simulink model "3DoFManipulator_SIMULATION"  (R2023b)
settings: Solver=ode45  StartTime=0.0  StopTime=10  RelTol=1e-3
undefined symbols (not defined in the file): X, Y, Z
libraries: sm_lib x10, nesl_utility x7, slpidlib x6, robotmaniplib x2
settings Model: Creator=nicog  LastModifiedBy=nicog

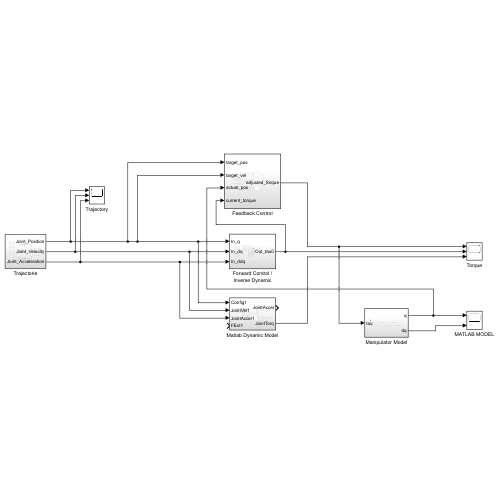
[thumbnail: Simulink's stored preview of the top-level diagram]
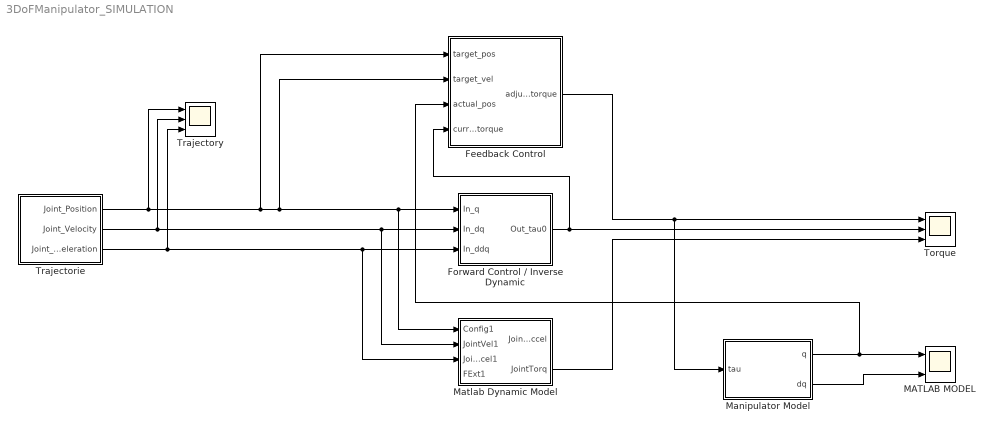
== system 3DoFManipulator_SIMULATION ==
  Feedback Control : Subsystem
  Forward Control / Inverse Dynamic : Subsystem
  MATLAB MODEL : Scope  NumInputPorts=2
  Manipulator Model : Subsystem
  Matlab Dynamic Model : Subsystem
  Torque : Scope  NumInputPorts=3
  Trajectorie : Subsystem
  Trajectory : Scope  NumInputPorts=3
  wires:
  Trajectorie/2(Joint_Velocity) -> Forward Control / Inverse Dynamic/2(In_dq), Matlab Dynamic Model/2(JointVel1), Trajectory/2
  Trajectorie/1(Joint_Position) -> Trajectory/1, Feedback Control/1(target_pos), Feedback Control/2(target_vel), Forward Control / Inverse Dynamic/1(In_q), Matlab Dynamic Model/1(Config1)
  Matlab Dynamic Model/2(JointTorq) -> Torque/3
  Trajectorie/3(Joint_Acceleration) -> Forward Control / Inverse Dynamic/3(In_ddq), Matlab Dynamic Model/3(JointAccel1), Trajectory/3
  Forward Control / Inverse Dynamic/1(Out_tau0) -> Feedback Control/4(current_torque), Torque/2
  Manipulator Model/1(q) -> Feedback Control/3(actual_pos), MATLAB MODEL/1
  Feedback Control/1(adjusted_torque) -> Manipulator Model/1(tau), Torque/1
  Manipulator Model/2(dq) -> MATLAB MODEL/2

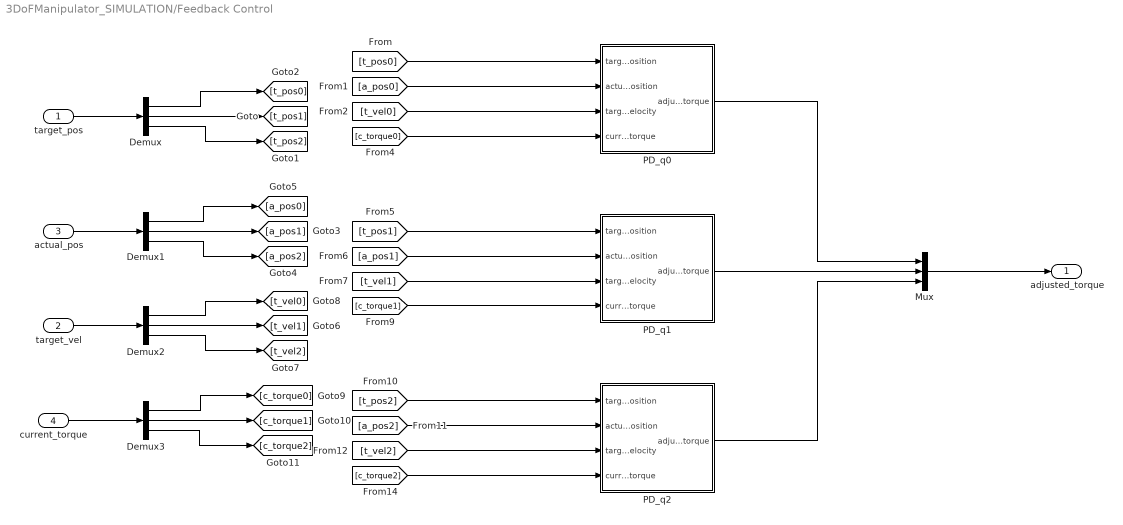
== system 3DoFManipulator_SIMULATION/Feedback Control ==
  target_pos : Inport
  target_vel : Inport  Port=2
  actual_pos : Inport  Port=3
  current_torque : Inport  Port=4
  Demux{,1..3} (4 alike) : Demux  Outputs=3
  Mux : Mux  Inputs=3
  PD_q0 : Subsystem
  PD_q1 : Subsystem
  PD_q2 : Subsystem
  adjusted_torque : Outport
  wires:
  target_pos/1 -> Demux/1
  actual_pos/1 -> Demux1/1
  target_vel/1 -> Demux2/1
  Demux/1 -> [t_pos0]
  Demux/2 -> [t_pos1]
  Demux/3 -> [t_pos2]
  Demux1/1 -> [a_pos0]
  Demux1/2 -> [a_pos1]
  Demux1/3 -> [a_pos2]
  Demux2/1 -> [t_vel0]
  Demux2/2 -> [t_vel1]
  Demux2/3 -> [t_vel2]
  [t_pos0] -> PD_q0/1(target position)
  [a_pos0] -> PD_q0/2(actual position)
  [t_vel0] -> PD_q0/3(target velocity)
  [c_torque0] -> PD_q0/4(current torque)
  Mux/1 -> adjusted_torque/1
  [c_torque1] -> PD_q1/4(current torque)
  [a_pos1] -> PD_q1/2(actual position)
  [t_vel1] -> PD_q1/3(target velocity)
  [t_pos1] -> PD_q1/1(target position)
  [c_torque2] -> PD_q2/4(current torque)
  [a_pos2] -> PD_q2/2(actual position)
  [t_vel2] -> PD_q2/3(target velocity)
  [t_pos2] -> PD_q2/1(target position)
  PD_q1/1(adjusted_torque) -> Mux/2
  PD_q2/1(adjusted_torque) -> Mux/3
  current_torque/1 -> Demux3/1
  Demux3/1 -> [c_torque0]
  Demux3/2 -> [c_torque1]
  Demux3/3 -> [c_torque2]
  PD_q0/1(adjusted_torque) -> Mux/1

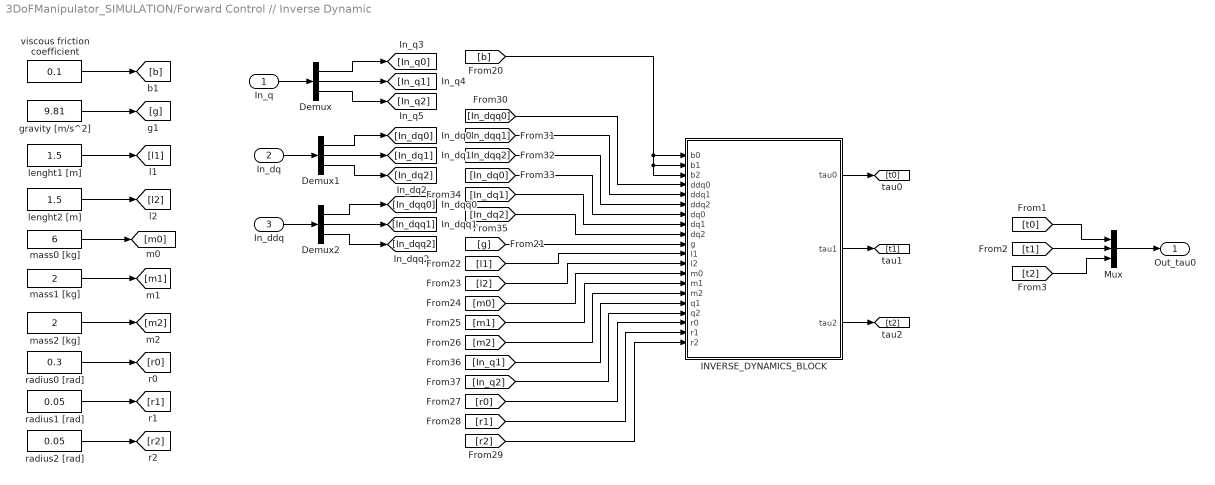
== system 3DoFManipulator_SIMULATION/Forward Control // Inverse Dynamic ==
  In_q : Inport
  In_dq : Inport  Port=2
  In_ddq : Inport  Port=3
  Demux : Demux  Outputs=3
  Demux1 : Demux  Outputs=3
  Demux2 : Demux  Outputs=3
  INVERSE_DYNAMICS_BLOCK : MATLAB Function  TreatAsAtomicUnit=on
  Mux : Mux  Inputs=3
  "gravity [m/s^2] " : Constant  Value=9.81
  lenght1 [m] : Constant  Value=1.5
  lenght2 [m] : Constant  Value=1.5
  mass0 [kg] : Constant  Value=6
  mass1 [kg] : Constant  Value=2
  mass2 [kg] : Constant  Value=2
  radius0 [rad] : Constant  Value=0.3
  radius1 [rad] : Constant  Value=0.05
  radius2 [rad] : Constant  Value=0.05
  viscous friction coefficient : Constant  Value=0.1
  Out_tau0 : Outport
  wires:
  [r2] -> INVERSE_DYNAMICS_BLOCK/20(r2)
  [g] -> INVERSE_DYNAMICS_BLOCK/10(g)
  [r0] -> INVERSE_DYNAMICS_BLOCK/18(r0)
  [b] -> INVERSE_DYNAMICS_BLOCK/2(b1), INVERSE_DYNAMICS_BLOCK/3(b2), INVERSE_DYNAMICS_BLOCK/1(b0)
  [l1] -> INVERSE_DYNAMICS_BLOCK/11(l1)
  [m1] -> INVERSE_DYNAMICS_BLOCK/14(m1)
  [m2] -> INVERSE_DYNAMICS_BLOCK/15(m2)
  [m0] -> INVERSE_DYNAMICS_BLOCK/13(m0)
  [r1] -> INVERSE_DYNAMICS_BLOCK/19(r1)
  [l2] -> INVERSE_DYNAMICS_BLOCK/12(l2)
  In_q/1 -> Demux/1
  In_dq/1 -> Demux1/1
  In_ddq/1 -> Demux2/1
  Mux/1 -> Out_tau0/1
  radius0 [rad]/1 -> [r0]
  radius2 [rad]/1 -> [r2]
  lenght2 [m]/1 -> [l2]
  viscous friction coefficient/1 -> [b]
  radius1 [rad]/1 -> [r1]
  lenght1 [m]/1 -> [l1]
  mass0 [kg]/1 -> [m0]
  mass1 [kg]/1 -> [m1]
  mass2 [kg]/1 -> [m2]
  "gravity [m/s^2] "/1 -> [g]
  INVERSE_DYNAMICS_BLOCK/3(tau2) -> [t2]
  [t0] -> Mux/1
  [t1] -> Mux/2
  [t2] -> Mux/3
  Demux2/1 -> [In_dqq0]
  Demux2/2 -> [In_dqq1]
  Demux2/3 -> [In_dqq2]
  Demux1/2 -> [In_dq1]
  Demux1/1 -> [In_dq0]
  Demux1/3 -> [In_dq2]
  Demux/2 -> [In_q1]
  Demux/1 -> [In_q0]
  Demux/3 -> [In_q2]
  [In_dqq0] -> INVERSE_DYNAMICS_BLOCK/4(ddq0)
  [In_dqq1] -> INVERSE_DYNAMICS_BLOCK/5(ddq1)
  [In_dqq2] -> INVERSE_DYNAMICS_BLOCK/6(ddq2)
  [In_dq0] -> INVERSE_DYNAMICS_BLOCK/7(dq0)
  [In_dq1] -> INVERSE_DYNAMICS_BLOCK/8(dq1)
  [In_dq2] -> INVERSE_DYNAMICS_BLOCK/9(dq2)
  [In_q1] -> INVERSE_DYNAMICS_BLOCK/16(q1)
  [In_q2] -> INVERSE_DYNAMICS_BLOCK/17(q2)
  INVERSE_DYNAMICS_BLOCK/2(tau1) -> [t1]
  INVERSE_DYNAMICS_BLOCK/1(tau0) -> [t0]

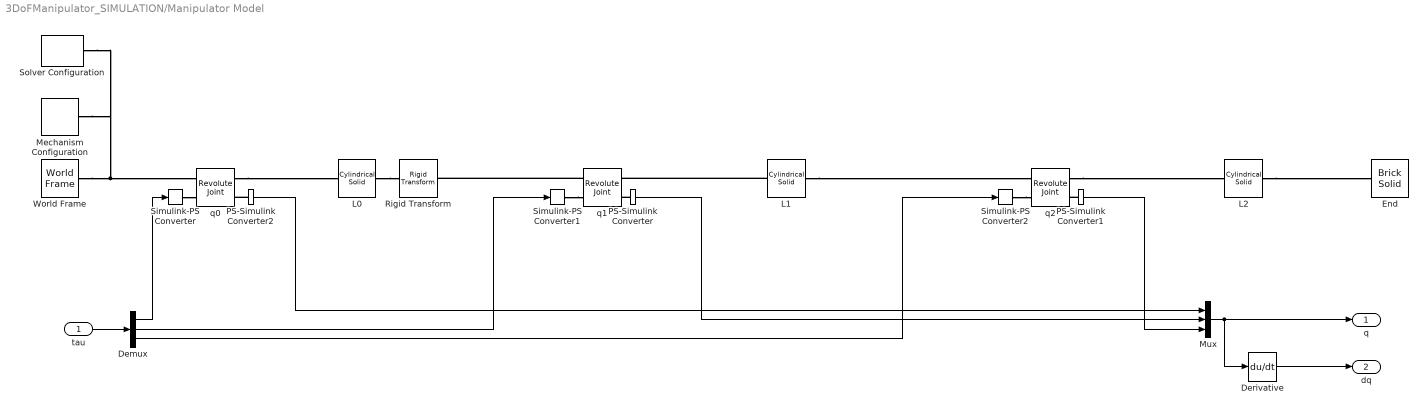
== system 3DoFManipulator_SIMULATION/Manipulator Model ==
  tau : Inport
  " L1" : sm_lib/Body Elements/Cylindrical Solid  GraphicAmbientColor=[0.15 0.15 0.15 1.0]  BasedOnType=Density  CenterOfMass=[0 0 0]  CenterOfMassUnits=m  GraphicDiffuseColor=[0.0 0.0 1.0]  CylinderLength=1.5  CylinderLengthUnits=m  CylinderRadius=0.05  CylinderRadiusUnits=m  Density=1000  DensityUnits=kg/m^3  DoExposeReferenceFrame=off  GraphicEmissiveColor=[0.0 0.0 0.0 1.0]  ExportEntireGeometry=off  SerializedFrames=<Frames><Frame><Id>Frame1</Id><Value><Name>F1</Name><Origin><Source>GeometricFeature</Source><FeatureName>bottom surface</FeatureName></Origin><PrimaryAxis><DefinedDirection>+X</DefinedDirection><Source>ReferenceFrame</Source><SourceDirection>+Z</SourceDirection><FeatureName></FeatureName></PrimaryAxis><SecondaryAxis><DefinedDirection>+Y</DefinedDirection><Source>ReferenceFrame</Source><SourceDirection>+X</SourceDirection><FeatureName></FeatureName></SecondaryAxis></Value></Frame><Frame><Id>Frame2</Id><Value><Name>F2</Name><Origin><Source>GeometricFeature</Source><FeatureName>top surface</FeatureName></Origin><PrimaryAxis><DefinedDirection>+X</DefinedDirection><Source>ReferenceFrame</Source><SourceDirection>+Z</SourceDirection><FeatureName></FeatureName></PrimaryAxis><SecondaryAxis><DefinedDirection>+Y</DefinedDirection><Source>ReferenceFrame</Source><SourceDirection>+X</SourceDirection><FeatureName></FeatureName></SecondaryAxis></Value></Frame></Frames>  MarkerShape=Sphere  MarkerSize=10  GraphicType=FromGeometry  InertiaType=PointMass  Mass=2  MassUnits=kg  MomentsOfInertia=[1 1 1]  MomentsOfInertiaUnits=kg*m^2  GraphicOpacity=1.0  ProductsOfInertia=[0 0 0]  ProductsOfInertiaUnits=kg*m^2  GraphicShininess=75  GraphicSpecularColor=[0.5 0.5 0.5 1.0]  GraphicVisPropType=SimpleVisualProperties
  Demux : Demux  Outputs=3
  Derivative : Derivative
  End : sm_lib/Body Elements/Brick Solid  GraphicAmbientColor=[0.15 0.15 0.15 1.0]  BasedOnType=Density  BrickDimensions=[1 1 1]  BrickDimensionsUnits=cm  CenterOfMass=[0 0 0]  CenterOfMassUnits=m  GraphicDiffuseColor=[1.0 0.0 0.4]  Density=1000  DensityUnits=kg/m^3  DoExposeReferenceFrame=on  GraphicEmissiveColor=[0.0 0.0 0.0 1.0]  ExportEntireGeometry=off  SerializedFrames=<Frames/>  MarkerShape=Sphere  MarkerSize=10  GraphicType=FromGeometry  InertiaType=PointMass  Mass=1  MassUnits=g  MomentsOfInertia=[1 1 1]  MomentsOfInertiaUnits=kg*m^2  GraphicOpacity=1.0  ProductsOfInertia=[0 0 0]  ProductsOfInertiaUnits=kg*m^2  GraphicShininess=75  GraphicSpecularColor=[0.5 0.5 0.5 1.0]  GraphicVisPropType=SimpleVisualProperties
  L0 : sm_lib/Body Elements/Cylindrical Solid  GraphicAmbientColor=[0.15 0.15 0.15 1.0]  BasedOnType=Density  CenterOfMass=[0 0 0]  CenterOfMassUnits=m  GraphicDiffuseColor=[1.0 1.0 0.0]  CylinderLength=0.5  CylinderLengthUnits=m  CylinderRadius=0.3  CylinderRadiusUnits=m  Density=1000  DensityUnits=kg/m^3  DoExposeReferenceFrame=off  GraphicEmissiveColor=[0.0 0.0 0.0 1.0]  ExportEntireGeometry=off  SerializedFrames=<Frames><Frame><Id>Frame1</Id><Value><Name>Bottom</Name><Origin><Source>GeometricFeature</Source><FeatureName>bottom surface</FeatureName></Origin><PrimaryAxis><DefinedDirection>+Z</DefinedDirection><Source>ReferenceFrame</Source><SourceDirection>+Z</SourceDirection><FeatureName></FeatureName></PrimaryAxis><SecondaryAxis><DefinedDirection>+X</DefinedDirection><Source>ReferenceFrame</Source><SourceDirection>+X</SourceDirection><FeatureName></FeatureName></SecondaryAxis></Value></Frame><Frame><Id>Frame2</Id><Value><Name>Top</Name><Origin><Source>GeometricFeature</Source><FeatureName>top surface</FeatureName></Origin><PrimaryAxis><DefinedDirection>+Z</DefinedDirection><Source>ReferenceFrame</Source><SourceDirection>+Z</SourceDirection><FeatureName></FeatureName></PrimaryAxis><SecondaryAxis><DefinedDirection>+X</DefinedDirection><Source>ReferenceFrame</Source><SourceDirection>+X</SourceDirection><FeatureName></FeatureName></SecondaryAxis></Value></Frame></Frames>  MarkerShape=Sphere  MarkerSize=10  GraphicType=FromGeometry  InertiaType=PointMass  Mass=6  MassUnits=kg  MomentsOfInertia=[1 1 1]  MomentsOfInertiaUnits=kg*m^2  GraphicOpacity=1.0  ProductsOfInertia=[0 0 0]  ProductsOfInertiaUnits=kg*m^2  GraphicShininess=75  GraphicSpecularColor=[0.5 0.5 0.5 1.0]  GraphicVisPropType=SimpleVisualProperties
  L2 : sm_lib/Body Elements/Cylindrical Solid  GraphicAmbientColor=[0.15 0.15 0.15 1.0]  BasedOnType=Density  CenterOfMass=[0 0 0]  CenterOfMassUnits=m  GraphicDiffuseColor=[1.0 0.6 0.0]  CylinderLength=1.5  CylinderLengthUnits=m  CylinderRadius=0.05  CylinderRadiusUnits=m  Density=1000  DensityUnits=kg/m^3  DoExposeReferenceFrame=off  GraphicEmissiveColor=[0.0 0.0 0.0 1.0]  ExportEntireGeometry=off  SerializedFrames=<Frames><Frame><Id>Frame1</Id><Value><Name>F1</Name><Origin><Source>GeometricFeature</Source><FeatureName>bottom surface</FeatureName></Origin><PrimaryAxis><DefinedDirection>+X</DefinedDirection><Source>ReferenceFrame</Source><SourceDirection>+Z</SourceDirection><FeatureName></FeatureName></PrimaryAxis><SecondaryAxis><DefinedDirection>+Y</DefinedDirection><Source>ReferenceFrame</Source><SourceDirection>+X</SourceDirection><FeatureName></FeatureName></SecondaryAxis></Value></Frame><Frame><Id>Frame2</Id><Value><Name>F2</Name><Origin><Source>GeometricFeature</Source><FeatureName>top surface</FeatureName></Origin><PrimaryAxis><DefinedDirection>+X</DefinedDirection><Source>ReferenceFrame</Source><SourceDirection>+Z</SourceDirection><FeatureName></FeatureName></PrimaryAxis><SecondaryAxis><DefinedDirection>+Y</DefinedDirection><Source>ReferenceFrame</Source><SourceDirection>+X</SourceDirection><FeatureName></FeatureName></SecondaryAxis></Value></Frame></Frames>  MarkerShape=Sphere  MarkerSize=10  GraphicType=FromGeometry  InertiaType=PointMass  Mass=2  MassUnits=kg  MomentsOfInertia=[1 1 1]  MomentsOfInertiaUnits=kg*m^2  GraphicOpacity=1.0  ProductsOfInertia=[0 0 0]  ProductsOfInertiaUnits=kg*m^2  GraphicShininess=75  GraphicSpecularColor=[0.5 0.5 0.5 1.0]  GraphicVisPropType=SimpleVisualProperties
  Mechanism Configuration : sm_lib/Utilities/Mechanism Configuration  UniformGravity=Constant  GravityVector=[0 0 -9.80665]  GravityVectorUnits=m/s^2  LinearizationDelta=0.001  JointModeTransitionNonlinearIterations=2
  Mux : Mux  Inputs=3
  PS-Simulink Converter : nesl_utility/PS-Simulink Converter  PhysicalDomain=network_engine_domain  SubClassName=ps_output  LeftPortType=input  RightPortType=output  PseudoPeriodic=off  Frequencies=[]  VectorFormat=inherit  Unit=inherit  AffineConversion=off
  PS-Simulink Converter1 : nesl_utility/PS-Simulink Converter  PhysicalDomain=network_engine_domain  SubClassName=ps_output  LeftPortType=input  RightPortType=output  PseudoPeriodic=off  Frequencies=[]  VectorFormat=inherit  Unit=inherit  AffineConversion=off
  PS-Simulink Converter2 : nesl_utility/PS-Simulink Converter  PhysicalDomain=network_engine_domain  SubClassName=ps_output  LeftPortType=input  RightPortType=output  PseudoPeriodic=off  Frequencies=[]  VectorFormat=inherit  Unit=inherit  AffineConversion=off
  Rigid Transform : sm_lib/Frames and Transforms/Rigid Transform  TranslationMethod=None  TranslationStandardOffset=0  TranslationStandardOffsetUnits=m  TranslationStandardAxis=+Z  TranslationCartesianOffset=[0 0 0]  TranslationCartesianOffsetUnits=m  TranslationROffset=0  TranslationROffsetUnits=m  TranslationZOffset=0  TranslationZOffsetUnits=m  TranslationThetaOffset=0  TranslationThetaOffsetUnits=deg  RotationMethod=RotationSequence  RotationAngleUnits=rad  RotationStandardAxis=+X  RotationAngle=pi/2  RotationArbitraryAxis=[0 0 1]  FollAlignAxisA=+X  BaseAlignAxisA=+Y  FollAlignAxisB=+Y  BaseAlignAxisB=+Z  RotationSequenceAxes=FollowerAxes  RotationSequence=XZX  RotationSequenceAngles=[90 0 0]  RotationSequenceAnglesUnits=deg  RotationMatrix=[1 0 0; 0 1 0; 0 0 1]  Quaternion=[1 0 0 0]
  Simulink-PS Converter : nesl_utility/Simulink-PS Converter  PhysicalDomain=network_engine_domain  SubClassName=ps_input  LeftPortType=input  RightPortType=output  PseudoPeriodic=off  Frequencies=[]  NoiseDistribution=none  NoiseParameters=[]  Unit=N*m  AffineConversion=off  FilteringAndDerivatives=provide  SimscapeFilterOrder=2  InputFilterTimeConstant=0.001  UdotUserProvided=0
  Simulink-PS Converter1 : nesl_utility/Simulink-PS Converter  PhysicalDomain=network_engine_domain  SubClassName=ps_input  LeftPortType=input  RightPortType=output  PseudoPeriodic=off  Frequencies=[]  NoiseDistribution=none  NoiseParameters=[]  Unit=N*m  AffineConversion=off  FilteringAndDerivatives=provide  SimscapeFilterOrder=2  InputFilterTimeConstant=0.001  UdotUserProvided=0
  Simulink-PS Converter2 : nesl_utility/Simulink-PS Converter  PhysicalDomain=network_engine_domain  SubClassName=ps_input  LeftPortType=input  RightPortType=output  PseudoPeriodic=off  Frequencies=[]  NoiseDistribution=none  NoiseParameters=[]  Unit=N*m  AffineConversion=off  FilteringAndDerivatives=provide  SimscapeFilterOrder=2  InputFilterTimeConstant=0.001  UdotUserProvided=0
  Solver Configuration : nesl_utility/Solver Configuration  PhysicalDomain=network_engine_domain  SubClassName=solver  LeftPortType=input  RightPortType=generic  Tones=[]  Harmonics=[]  SimulateNoise=off  Profile=off  UseLocalSampling=off  EnableSwitchedLinearOptims=on  FrequencyDomain=off  UseCCode=off  RelTol=0.001  AbsTol=0.001  MinStep=1e-09  ToWorkspace=off  RevertToSquareIcSolve=off  NumHomotopyIterations=100  PhasorMode=off  PhasorModeNumHarmonics=1  ConsistencySolver=NEWTON_XTOL_AFTER_FTOL  IndexReductionMethod=DerivativeReplacement  DoDC=off  ResidualTolerance=1e-09  ConsistencyTolSource=GLOBAL  ConsistencyAbsTol=0.001  ConsistencyRelTol=0.001  ConsistencyTolFactor=0.001  UseLocalSolver=off  LocalSolverChoice=NE_BACKWARD_EULER_ADVANCER  ResolveIndetEquations=on  FunctionEvalNumThread=1  LocalSolverSampleTime=0.001  DoFixedCost=off  MaxNonlinIter=3  MaxModeIter=2  ComputeImpulses=off  ImpulseIterations=2  LinearAlgebra=auto  LinearAlgebraNumThread=0  EquationFormulation=NE_TIME_EF  DelaysMemoryBudget=1024  AutomaticFiltering=on  FilteringTimeConstant=0.001  PartitionStorageMethod=AS_NEEDED  PartitionMemoryBudget=1024  PartitionMethod=ROBUST  MultibodyUseLocalSolver=off  MultibodyLocalSolverChoice=ODE1  MultibodyLocalSolverSampleTime=0.001
  World Frame : sm_lib/Frames and Transforms/World Frame
  q0 : sm_lib/Joints/Revolute Joint  JointMode=Normal  SenseConstraintForce=off  SenseConstraintForceX=off  SenseConstraintForceY=off  SenseConstraintForceZ=off  SenseConstraintTorque=off  SenseConstraintTorqueX=off  SenseConstraintTorqueY=off  SenseConstraintTorqueZ=off  SenseTotalForce=off  SenseTotalForceX=off  SenseTotalForceY=off  SenseTotalForceZ=off  SenseTotalTorque=off  SenseTotalTorqueX=off  SenseTotalTorqueY=off  SenseTotalTorqueZ=off  CompositeWrenchDir=FollowerOnBase  CompositeWrenchFrame=BaseFrame  EquilibriumPosition=0  EquilibriumPositionUnits=deg  SpringStiffness=0  SpringStiffnessUnits=N*m/deg  DampingCoefficient=0  DampingCoefficientUnits=N*m/(deg/s)  TorqueActuationMode=InputTorque  MotionActuationMode=ComputedMotion  SensePosition=on  SenseVelocity=off  SenseAcceleration=off  SenseTorqueForce=off  SenseLowerLimitTorqueForce=off  SenseUpperLimitTorqueForce=off  LowerLimitSpecify=on  LowerLimitBound=-180  LowerLimitBoundUnits=deg  LowerLimitStiffness=1e4  LowerLimitStiffnessUnits=N*m/deg  LowerLimitDamping=10  LowerLimitDampingUnits=N*m/(deg/s)  LowerLimitTransitionRegionWidth=0.1  LowerLimitTransitionRegionWidthUnits=deg  UpperLimitSpecify=on  UpperLimitBound=180  UpperLimitBoundUnits=deg  UpperLimitStiffness=1e4  UpperLimitStiffnessUnits=N*m/deg  UpperLimitDamping=10  UpperLimitDampingUnits=N*m/(deg/s)  UpperLimitTransitionRegionWidth=0.1  UpperLimitTransitionRegionWidthUnits=deg  PositionTargetSpecify=off  PositionTargetPriority=High  PositionTargetValue=0  PositionTargetValueUnits=deg  VelocityTargetSpecify=off  VelocityTargetPriority=High  VelocityTargetValue=0  VelocityTargetValueUnits=deg/s
  q1 : sm_lib/Joints/Revolute Joint  JointMode=Normal  SenseConstraintForce=off  SenseConstraintForceX=off  SenseConstraintForceY=off  SenseConstraintForceZ=off  SenseConstraintTorque=off  SenseConstraintTorqueX=off  SenseConstraintTorqueY=off  SenseConstraintTorqueZ=off  SenseTotalForce=off  SenseTotalForceX=off  SenseTotalForceY=off  SenseTotalForceZ=off  SenseTotalTorque=off  SenseTotalTorqueX=off  SenseTotalTorqueY=off  SenseTotalTorqueZ=off  CompositeWrenchDir=FollowerOnBase  CompositeWrenchFrame=BaseFrame  EquilibriumPosition=0  EquilibriumPositionUnits=deg  SpringStiffness=0  SpringStiffnessUnits=N*m/deg  DampingCoefficient=0  DampingCoefficientUnits=N*m/(deg/s)  TorqueActuationMode=InputTorque  MotionActuationMode=ComputedMotion  SensePosition=on  SenseVelocity=off  SenseAcceleration=off  SenseTorqueForce=off  SenseLowerLimitTorqueForce=off  SenseUpperLimitTorqueForce=off  LowerLimitSpecify=on  LowerLimitBound=0  LowerLimitBoundUnits=deg  LowerLimitStiffness=1e4  LowerLimitStiffnessUnits=N*m/deg  LowerLimitDamping=10  LowerLimitDampingUnits=N*m/(deg/s)  LowerLimitTransitionRegionWidth=0.1  LowerLimitTransitionRegionWidthUnits=deg  UpperLimitSpecify=on  UpperLimitBound=120  UpperLimitBoundUnits=deg  UpperLimitStiffness=1e4  UpperLimitStiffnessUnits=N*m/deg  UpperLimitDamping=10  UpperLimitDampingUnits=N*m/(deg/s)  UpperLimitTransitionRegionWidth=0.1  UpperLimitTransitionRegionWidthUnits=deg  PositionTargetSpecify=off  PositionTargetPriority=High  PositionTargetValue=0  PositionTargetValueUnits=deg  VelocityTargetSpecify=off  VelocityTargetPriority=High  VelocityTargetValue=0  VelocityTargetValueUnits=deg/s
  q2 : sm_lib/Joints/Revolute Joint  JointMode=Normal  SenseConstraintForce=off  SenseConstraintForceX=off  SenseConstraintForceY=off  SenseConstraintForceZ=off  SenseConstraintTorque=off  SenseConstraintTorqueX=off  SenseConstraintTorqueY=off  SenseConstraintTorqueZ=off  SenseTotalForce=off  SenseTotalForceX=off  SenseTotalForceY=off  SenseTotalForceZ=off  SenseTotalTorque=off  SenseTotalTorqueX=off  SenseTotalTorqueY=off  SenseTotalTorqueZ=off  CompositeWrenchDir=FollowerOnBase  CompositeWrenchFrame=BaseFrame  EquilibriumPosition=0  EquilibriumPositionUnits=deg  SpringStiffness=0  SpringStiffnessUnits=N*m/deg  DampingCoefficient=0  DampingCoefficientUnits=N*m/(deg/s)  TorqueActuationMode=InputTorque  MotionActuationMode=ComputedMotion  SensePosition=on  SenseVelocity=off  SenseAcceleration=off  SenseTorqueForce=off  SenseLowerLimitTorqueForce=off  SenseUpperLimitTorqueForce=off  LowerLimitSpecify=on  LowerLimitBound=-120  LowerLimitBoundUnits=deg  LowerLimitStiffness=1e4  LowerLimitStiffnessUnits=N*m/deg  LowerLimitDamping=10  LowerLimitDampingUnits=N*m/(deg/s)  LowerLimitTransitionRegionWidth=0.1  LowerLimitTransitionRegionWidthUnits=deg  UpperLimitSpecify=on  UpperLimitBound=0  UpperLimitBoundUnits=deg  UpperLimitStiffness=1e4  UpperLimitStiffnessUnits=N*m/deg  UpperLimitDamping=10  UpperLimitDampingUnits=N*m/(deg/s)  UpperLimitTransitionRegionWidth=0.1  UpperLimitTransitionRegionWidthUnits=deg  PositionTargetSpecify=off  PositionTargetPriority=High  PositionTargetValue=0  PositionTargetValueUnits=deg  VelocityTargetSpecify=off  VelocityTargetPriority=High  VelocityTargetValue=0  VelocityTargetValueUnits=deg/s
  q : Outport
  dq : Outport  Port=2
  wires:
  Demux/3 -> Simulink-PS Converter2/1
  Demux/1 -> Simulink-PS Converter/1
  PS-Simulink Converter1/1 -> Mux/3
  Demux/2 -> Simulink-PS Converter1/1
  PS-Simulink Converter/1 -> Mux/2
  PS-Simulink Converter2/1 -> Mux/1
  tau/1 -> Demux/1
  Mux/1 -> q/1, Derivative/1
  Derivative/1 -> dq/1
  connections:
  PS-Simulink Converter2/LConn1 -- q0/RConn2
  " L1"/RConn1 -- q2/LConn1
  q1/LConn1 -- Rigid Transform/RConn1
  q0/RConn1 -- L0/LConn1
  World Frame/RConn1 -- Solver Configuration/RConn1 -- Mechanism Configuration/RConn1 -- q0/LConn1
  q2/RConn1 -- L2/LConn1
  " L1"/LConn1 -- q1/RConn1
  L0/RConn1 -- Rigid Transform/LConn1
  Simulink-PS Converter/RConn1 -- q0/LConn2
  PS-Simulink Converter1/LConn1 -- q2/RConn2
  Simulink-PS Converter1/RConn1 -- q1/LConn2
  PS-Simulink Converter/LConn1 -- q1/RConn2
  Simulink-PS Converter2/RConn1 -- q2/LConn2
  L2/RConn1 -- End/RConn1

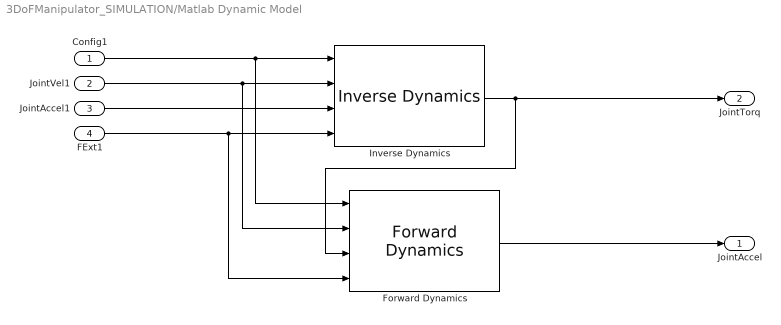
== system 3DoFManipulator_SIMULATION/Matlab Dynamic Model ==
  Config1 : Inport
  JointVel1 : Inport  Port=2
  JointAccel1 : Inport  Port=3
  FExt1 : Inport  Port=4
  Forward Dynamics : robotmaniplib/Forward Dynamics  RigidBodyTree=ArmModel  SimulateUsing=Interpreted execution
  Inverse Dynamics : robotmaniplib/Inverse Dynamics  RigidBodyTree=ArmModel  SimulateUsing=Interpreted execution
  JointAccel : Outport
  JointTorq : Outport  Port=2
  wires:
  Config1/1 -> Forward Dynamics/1, Inverse Dynamics/1
  Forward Dynamics/1 -> JointAccel/1
  FExt1/1 -> Forward Dynamics/4, Inverse Dynamics/4
  JointVel1/1 -> Forward Dynamics/2, Inverse Dynamics/2
  JointAccel1/1 -> Inverse Dynamics/3
  Inverse Dynamics/1 -> JointTorq/1, Forward Dynamics/3

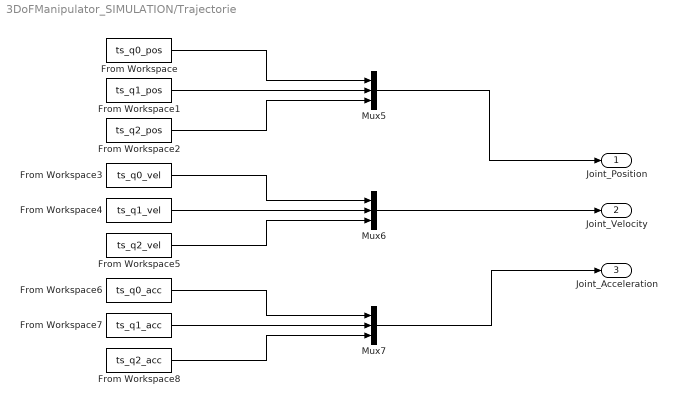
== system 3DoFManipulator_SIMULATION/Trajectorie ==
  From Workspace : FromWorkspace  VariableName=ts_q0_pos
  From Workspace1 : FromWorkspace  VariableName=ts_q1_pos
  From Workspace2 : FromWorkspace  VariableName=ts_q2_pos
  From Workspace3 : FromWorkspace  VariableName=ts_q0_vel
  From Workspace4 : FromWorkspace  VariableName=ts_q1_vel
  From Workspace5 : FromWorkspace  VariableName=ts_q2_vel
  From Workspace6 : FromWorkspace  VariableName=ts_q0_acc
  From Workspace7 : FromWorkspace  VariableName=ts_q1_acc
  From Workspace8 : FromWorkspace  VariableName=ts_q2_acc
  Mux5 : Mux  Inputs=3
  Mux6 : Mux  Inputs=3
  Mux7 : Mux  Inputs=3
  Joint_Position : Outport
  Joint_Velocity : Outport  Port=2
  Joint_Acceleration : Outport  Port=3
  wires:
  From Workspace3/1 -> Mux6/1
  From Workspace2/1 -> Mux5/3
  From Workspace5/1 -> Mux6/3
  From Workspace4/1 -> Mux6/2
  From Workspace6/1 -> Mux7/1
  From Workspace8/1 -> Mux7/3
  From Workspace/1 -> Mux5/1
  From Workspace1/1 -> Mux5/2
  From Workspace7/1 -> Mux7/2
  Mux5/1 -> Joint_Position/1
  Mux7/1 -> Joint_Acceleration/1
  Mux6/1 -> Joint_Velocity/1

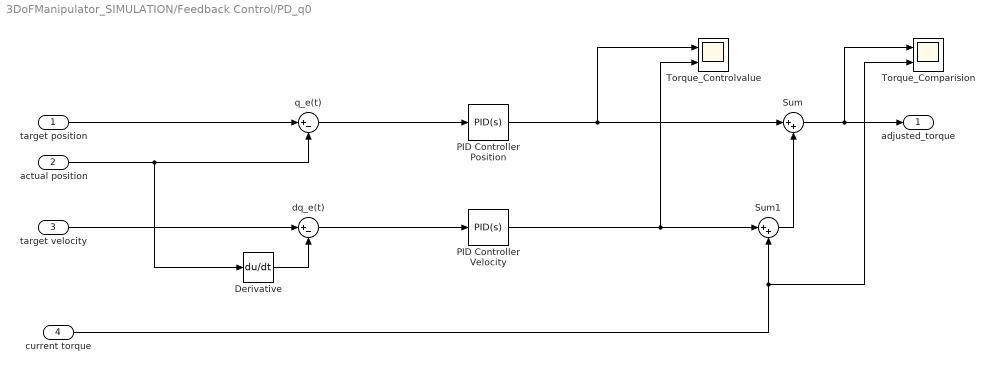
== system 3DoFManipulator_SIMULATION/Feedback Control/PD_q0 ==
  target position : Inport
  actual position : Inport  Port=2
  target velocity : Inport  Port=3
  current torque : Inport  Port=4
  Derivative : Derivative
  PID Controller Position : slpidlib/PID Controller  Controller=PID  Form=Parallel  TimeDomain=Continuous-time  UseExternalTs=off  SampleTime=-1  IntegratorMethod=Forward Euler  FilterMethod=Forward Euler  ControllerParametersSource=internal  P=1000  I=0  UseKiTs=off  D=50  N=100  UseFilter=on  TunerSelectOption=Transfer Function Based (PID Tuner App)  InitialConditionSource=internal  InitialConditionForIntegrator=0  InitialConditionForFilter=0  DifferentiatorICPrevScaledInput=0  ExternalReset=none  TrackingMode=off  Kt=1  LimitOutput=off  SatLimitsSource=internal  UpperSaturationLimit=inf  LowerSaturationLimit=-inf  LinearizeAsGain=on  AntiWindupMode=none  Kb=1  LimitIntegrator=off  UpperIntegratorSaturationLimit=inf  LowerIntegratorSaturationLimit=-inf  POutMin=[]  POutMax=[]  IOutMin=[]  IOutMax=[]  DOutMin=[]  DOutMax=[]  NOutMin=[]  NOutMax=[]  SumOutMin=[]  SumOutMax=[]  SaturationOutMin=[]  SaturationOutMax=[]  PParamMin=[]  PParamMax=[]  IParamMin=[]  IParamMax=[]  DParamMin=[]  DParamMax=[]  NParamMin=[]  NParamMax=[]  KbParamMin=[]  KbParamMax=[]  KtParamMin=[]  KtParamMax=[]  KbOutMin=[]  KbOutMax=[]  KtOutMin=[]  KtOutMax=[]  IntegratorOutMin=[]  IntegratorOutMax=[]  FilterOutMin=[]  FilterOutMax=[]  SumI1OutMin=[]  SumI1OutMax=[]  SumI2OutMin=[]  SumI2OutMax=[]  SumI3OutMin=[]  SumI3OutMax=[]  SumI4OutMin=[]  SumI4OutMax=[]  SumDOutMin=[]  SumDOutMax=[]  DifferentiatorOutMin=[]  DifferentiatorOutMax=[]  FilterDiffOutCoefMin=[]  FilterDiffOutCoefMax=[]  ReciprocalOutMin=[]  ReciprocalOutMax=[]  SumDenOutMin=[]  SumDenOutMax=[]  SumNumOutMin=[]  SumNumOutMax=[]  DivideOutMin=[]  DivideOutMax=[]  UdiffTsProdOutMin=[]  UdiffTsProdOutMax=[]  NTsProdOutMin=[]  NTsProdOutMax=[]  UintegralTsProdOutMin=[]  UintegralTsProdOutMax=[]  UngainTsProdOutMin=[]  UngainTsProdOutMax=[]  ClampingZeroOutDataTypeStr=Inherit: Inherit via back propagation  ClampingZeroOutMin=[]  ClampingZeroOutMax=[]  FilterDenConstantOutDataTypeStr=Inherit: Inherit via back propagation  FilterDenConstantOutMin=[]  FilterDenConstantOutMax=[]  PCopyOutDataTypeStr=Inherit: Inherit via back propagation  PCopyOutMin=[]  PCopyOutMax=[]  NCopyOutDataTypeStr=Inherit: Inherit via back propagation  NCopyOutMin=[]  NCopyOutMax=[]  IntegratorContinuousStateAttributes=''  IntegratorStateMustResolveToSignalObject=off  IntegratorRTWStateStorageClass=Auto  FilterContinuousStateAttributes=''  FilterStateMustResolveToSignalObject=off  FilterRTWStateStorageClass=Auto  ParallelPVariant=InternalParameters  IdealPVariant=Disabled  IVariant=InternalParameters  DVariant=InternalParameters  IntegratorVariant=Continuous  SatVariant=Disabled  AWVariant=Passthrough  PCopyVariant=Disabled  TRVariant=Disabled  FdbkBlocksVariant=Forward  IdealPFdbkVariant=Disabled  SatFdbkVariant=Disabled  DerivativeFilterVariant=ContFilter  NVariant=InternalParameters  NCopyVariant=Disabled  FilterICVariant=InternalICsFilter  IntegratorICVariant=InternalICs  ExternalResetVariant=Disabled  TRSumVariant=Passthrough  SumFdbkVariant=Disabled  SumVariant=Sum_PID  TsampFilterVariant=InternalTs  TsampNgainVariant=Passthrough  TsampIntegralVariant=Disabled_SignalSpec  ExternalSaturationOutDataTypeStr=Inherit: Same as second input
  PID Controller Velocity : slpidlib/PID Controller  Controller=PID  Form=Parallel  TimeDomain=Continuous-time  UseExternalTs=off  SampleTime=-1  IntegratorMethod=Forward Euler  FilterMethod=Forward Euler  ControllerParametersSource=internal  P=15  I=0  UseKiTs=off  D=1  N=100  UseFilter=on  TunerSelectOption=Transfer Function Based (PID Tuner App)  InitialConditionSource=internal  InitialConditionForIntegrator=0  InitialConditionForFilter=0  DifferentiatorICPrevScaledInput=0  ExternalReset=none  TrackingMode=off  Kt=1  LimitOutput=off  SatLimitsSource=internal  UpperSaturationLimit=inf  LowerSaturationLimit=-inf  LinearizeAsGain=on  AntiWindupMode=none  Kb=1  LimitIntegrator=off  UpperIntegratorSaturationLimit=inf  LowerIntegratorSaturationLimit=-inf  POutMin=[]  POutMax=[]  IOutMin=[]  IOutMax=[]  DOutMin=[]  DOutMax=[]  NOutMin=[]  NOutMax=[]  SumOutMin=[]  SumOutMax=[]  SaturationOutMin=[]  SaturationOutMax=[]  PParamMin=[]  PParamMax=[]  IParamMin=[]  IParamMax=[]  DParamMin=[]  DParamMax=[]  NParamMin=[]  NParamMax=[]  KbParamMin=[]  KbParamMax=[]  KtParamMin=[]  KtParamMax=[]  KbOutMin=[]  KbOutMax=[]  KtOutMin=[]  KtOutMax=[]  IntegratorOutMin=[]  IntegratorOutMax=[]  FilterOutMin=[]  FilterOutMax=[]  SumI1OutMin=[]  SumI1OutMax=[]  SumI2OutMin=[]  SumI2OutMax=[]  SumI3OutMin=[]  SumI3OutMax=[]  SumI4OutMin=[]  SumI4OutMax=[]  SumDOutMin=[]  SumDOutMax=[]  DifferentiatorOutMin=[]  DifferentiatorOutMax=[]  FilterDiffOutCoefMin=[]  FilterDiffOutCoefMax=[]  ReciprocalOutMin=[]  ReciprocalOutMax=[]  SumDenOutMin=[]  SumDenOutMax=[]  SumNumOutMin=[]  SumNumOutMax=[]  DivideOutMin=[]  DivideOutMax=[]  UdiffTsProdOutMin=[]  UdiffTsProdOutMax=[]  NTsProdOutMin=[]  NTsProdOutMax=[]  UintegralTsProdOutMin=[]  UintegralTsProdOutMax=[]  UngainTsProdOutMin=[]  UngainTsProdOutMax=[]  ClampingZeroOutDataTypeStr=Inherit: Inherit via back propagation  ClampingZeroOutMin=[]  ClampingZeroOutMax=[]  FilterDenConstantOutDataTypeStr=Inherit: Inherit via back propagation  FilterDenConstantOutMin=[]  FilterDenConstantOutMax=[]  PCopyOutDataTypeStr=Inherit: Inherit via back propagation  PCopyOutMin=[]  PCopyOutMax=[]  NCopyOutDataTypeStr=Inherit: Inherit via back propagation  NCopyOutMin=[]  NCopyOutMax=[]  IntegratorContinuousStateAttributes=''  IntegratorStateMustResolveToSignalObject=off  IntegratorRTWStateStorageClass=Auto  FilterContinuousStateAttributes=''  FilterStateMustResolveToSignalObject=off  FilterRTWStateStorageClass=Auto  ParallelPVariant=InternalParameters  IdealPVariant=Disabled  IVariant=InternalParameters  DVariant=InternalParameters  IntegratorVariant=Continuous  SatVariant=Disabled  AWVariant=Passthrough  PCopyVariant=Disabled  TRVariant=Disabled  FdbkBlocksVariant=Forward  IdealPFdbkVariant=Disabled  SatFdbkVariant=Disabled  DerivativeFilterVariant=ContFilter  NVariant=InternalParameters  NCopyVariant=Disabled  FilterICVariant=InternalICsFilter  IntegratorICVariant=InternalICs  ExternalResetVariant=Disabled  TRSumVariant=Passthrough  SumFdbkVariant=Disabled  SumVariant=Sum_PID  TsampFilterVariant=InternalTs  TsampNgainVariant=Passthrough  TsampIntegralVariant=Disabled_SignalSpec  ExternalSaturationOutDataTypeStr=Inherit: Same as second input
  Sum : Sum  Inputs=|++
  Sum1 : Sum  Inputs=|++
  Torque_Comparision : Scope  NumInputPorts=2
  Torque_Controlvalue : Scope  NumInputPorts=2
  dq_e(t) : Sum  Inputs=|+-
  q_e(t) : Sum  Inputs=|+-
  adjusted_torque : Outport
  wires:
  PID Controller Position/1 -> Sum/1, Torque_Controlvalue/1
  PID Controller Velocity/1 -> Torque_Controlvalue/2, Sum1/1
  dq_e(t)/1 -> PID Controller Velocity/1
  current torque/1 -> Torque_Comparision/2, Sum1/2
  q_e(t)/1 -> PID Controller Position/1
  actual position/1 -> Derivative/1, q_e(t)/2
  Sum1/1 -> Sum/2
  target position/1 -> q_e(t)/1
  Derivative/1 -> dq_e(t)/2
  Sum/1 -> Torque_Comparision/1, adjusted_torque/1
  target velocity/1 -> dq_e(t)/1

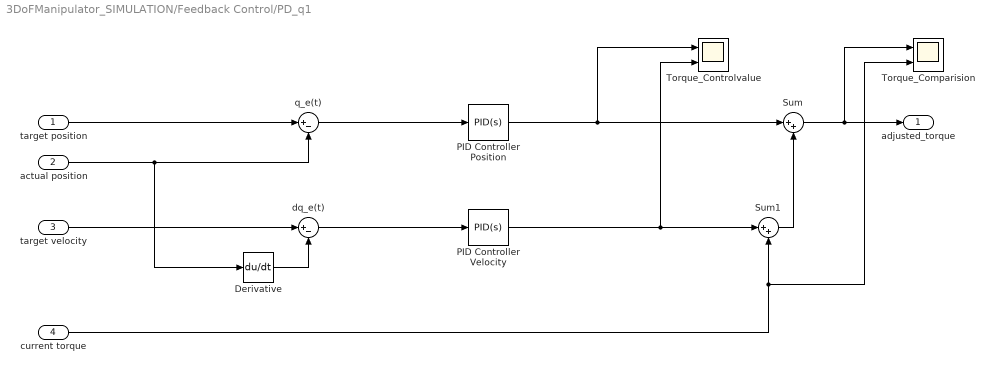
== system 3DoFManipulator_SIMULATION/Feedback Control/PD_q1 ==
  target position : Inport
  actual position : Inport  Port=2
  target velocity : Inport  Port=3
  current torque : Inport  Port=4
  Derivative : Derivative
  PID Controller Position : slpidlib/PID Controller  Controller=PID  Form=Parallel  TimeDomain=Continuous-time  UseExternalTs=off  SampleTime=-1  IntegratorMethod=Forward Euler  FilterMethod=Forward Euler  ControllerParametersSource=internal  P=300  I=0  UseKiTs=off  D=50  N=100  UseFilter=on  TunerSelectOption=Transfer Function Based (PID Tuner App)  InitialConditionSource=internal  InitialConditionForIntegrator=0  InitialConditionForFilter=0  DifferentiatorICPrevScaledInput=0  ExternalReset=none  TrackingMode=off  Kt=1  LimitOutput=off  SatLimitsSource=internal  UpperSaturationLimit=inf  LowerSaturationLimit=-inf  LinearizeAsGain=on  AntiWindupMode=none  Kb=1  LimitIntegrator=off  UpperIntegratorSaturationLimit=inf  LowerIntegratorSaturationLimit=-inf  POutMin=[]  POutMax=[]  IOutMin=[]  IOutMax=[]  DOutMin=[]  DOutMax=[]  NOutMin=[]  NOutMax=[]  SumOutMin=[]  SumOutMax=[]  SaturationOutMin=[]  SaturationOutMax=[]  PParamMin=[]  PParamMax=[]  IParamMin=[]  IParamMax=[]  DParamMin=[]  DParamMax=[]  NParamMin=[]  NParamMax=[]  KbParamMin=[]  KbParamMax=[]  KtParamMin=[]  KtParamMax=[]  KbOutMin=[]  KbOutMax=[]  KtOutMin=[]  KtOutMax=[]  IntegratorOutMin=[]  IntegratorOutMax=[]  FilterOutMin=[]  FilterOutMax=[]  SumI1OutMin=[]  SumI1OutMax=[]  SumI2OutMin=[]  SumI2OutMax=[]  SumI3OutMin=[]  SumI3OutMax=[]  SumI4OutMin=[]  SumI4OutMax=[]  SumDOutMin=[]  SumDOutMax=[]  DifferentiatorOutMin=[]  DifferentiatorOutMax=[]  FilterDiffOutCoefMin=[]  FilterDiffOutCoefMax=[]  ReciprocalOutMin=[]  ReciprocalOutMax=[]  SumDenOutMin=[]  SumDenOutMax=[]  SumNumOutMin=[]  SumNumOutMax=[]  DivideOutMin=[]  DivideOutMax=[]  UdiffTsProdOutMin=[]  UdiffTsProdOutMax=[]  NTsProdOutMin=[]  NTsProdOutMax=[]  UintegralTsProdOutMin=[]  UintegralTsProdOutMax=[]  UngainTsProdOutMin=[]  UngainTsProdOutMax=[]  ClampingZeroOutDataTypeStr=Inherit: Inherit via back propagation  ClampingZeroOutMin=[]  ClampingZeroOutMax=[]  FilterDenConstantOutDataTypeStr=Inherit: Inherit via back propagation  FilterDenConstantOutMin=[]  FilterDenConstantOutMax=[]  PCopyOutDataTypeStr=Inherit: Inherit via back propagation  PCopyOutMin=[]  PCopyOutMax=[]  NCopyOutDataTypeStr=Inherit: Inherit via back propagation  NCopyOutMin=[]  NCopyOutMax=[]  IntegratorContinuousStateAttributes=''  IntegratorStateMustResolveToSignalObject=off  IntegratorRTWStateStorageClass=Auto  FilterContinuousStateAttributes=''  FilterStateMustResolveToSignalObject=off  FilterRTWStateStorageClass=Auto  ParallelPVariant=InternalParameters  IdealPVariant=Disabled  IVariant=InternalParameters  DVariant=InternalParameters  IntegratorVariant=Continuous  SatVariant=Disabled  AWVariant=Passthrough  PCopyVariant=Disabled  TRVariant=Disabled  FdbkBlocksVariant=Forward  IdealPFdbkVariant=Disabled  SatFdbkVariant=Disabled  DerivativeFilterVariant=ContFilter  NVariant=InternalParameters  NCopyVariant=Disabled  FilterICVariant=InternalICsFilter  IntegratorICVariant=InternalICs  ExternalResetVariant=Disabled  TRSumVariant=Passthrough  SumFdbkVariant=Disabled  SumVariant=Sum_PID  TsampFilterVariant=InternalTs  TsampNgainVariant=Passthrough  TsampIntegralVariant=Disabled_SignalSpec  ExternalSaturationOutDataTypeStr=Inherit: Same as second input
  PID Controller Velocity : slpidlib/PID Controller  Controller=PID  Form=Parallel  TimeDomain=Continuous-time  UseExternalTs=off  SampleTime=-1  IntegratorMethod=Forward Euler  FilterMethod=Forward Euler  ControllerParametersSource=internal  P=10  I=0  UseKiTs=off  D=1  N=100  UseFilter=on  TunerSelectOption=Transfer Function Based (PID Tuner App)  InitialConditionSource=internal  InitialConditionForIntegrator=0  InitialConditionForFilter=0  DifferentiatorICPrevScaledInput=0  ExternalReset=none  TrackingMode=off  Kt=1  LimitOutput=off  SatLimitsSource=internal  UpperSaturationLimit=inf  LowerSaturationLimit=-inf  LinearizeAsGain=on  AntiWindupMode=none  Kb=1  LimitIntegrator=off  UpperIntegratorSaturationLimit=inf  LowerIntegratorSaturationLimit=-inf  POutMin=[]  POutMax=[]  IOutMin=[]  IOutMax=[]  DOutMin=[]  DOutMax=[]  NOutMin=[]  NOutMax=[]  SumOutMin=[]  SumOutMax=[]  SaturationOutMin=[]  SaturationOutMax=[]  PParamMin=[]  PParamMax=[]  IParamMin=[]  IParamMax=[]  DParamMin=[]  DParamMax=[]  NParamMin=[]  NParamMax=[]  KbParamMin=[]  KbParamMax=[]  KtParamMin=[]  KtParamMax=[]  KbOutMin=[]  KbOutMax=[]  KtOutMin=[]  KtOutMax=[]  IntegratorOutMin=[]  IntegratorOutMax=[]  FilterOutMin=[]  FilterOutMax=[]  SumI1OutMin=[]  SumI1OutMax=[]  SumI2OutMin=[]  SumI2OutMax=[]  SumI3OutMin=[]  SumI3OutMax=[]  SumI4OutMin=[]  SumI4OutMax=[]  SumDOutMin=[]  SumDOutMax=[]  DifferentiatorOutMin=[]  DifferentiatorOutMax=[]  FilterDiffOutCoefMin=[]  FilterDiffOutCoefMax=[]  ReciprocalOutMin=[]  ReciprocalOutMax=[]  SumDenOutMin=[]  SumDenOutMax=[]  SumNumOutMin=[]  SumNumOutMax=[]  DivideOutMin=[]  DivideOutMax=[]  UdiffTsProdOutMin=[]  UdiffTsProdOutMax=[]  NTsProdOutMin=[]  NTsProdOutMax=[]  UintegralTsProdOutMin=[]  UintegralTsProdOutMax=[]  UngainTsProdOutMin=[]  UngainTsProdOutMax=[]  ClampingZeroOutDataTypeStr=Inherit: Inherit via back propagation  ClampingZeroOutMin=[]  ClampingZeroOutMax=[]  FilterDenConstantOutDataTypeStr=Inherit: Inherit via back propagation  FilterDenConstantOutMin=[]  FilterDenConstantOutMax=[]  PCopyOutDataTypeStr=Inherit: Inherit via back propagation  PCopyOutMin=[]  PCopyOutMax=[]  NCopyOutDataTypeStr=Inherit: Inherit via back propagation  NCopyOutMin=[]  NCopyOutMax=[]  IntegratorContinuousStateAttributes=''  IntegratorStateMustResolveToSignalObject=off  IntegratorRTWStateStorageClass=Auto  FilterContinuousStateAttributes=''  FilterStateMustResolveToSignalObject=off  FilterRTWStateStorageClass=Auto  ParallelPVariant=InternalParameters  IdealPVariant=Disabled  IVariant=InternalParameters  DVariant=InternalParameters  IntegratorVariant=Continuous  SatVariant=Disabled  AWVariant=Passthrough  PCopyVariant=Disabled  TRVariant=Disabled  FdbkBlocksVariant=Forward  IdealPFdbkVariant=Disabled  SatFdbkVariant=Disabled  DerivativeFilterVariant=ContFilter  NVariant=InternalParameters  NCopyVariant=Disabled  FilterICVariant=InternalICsFilter  IntegratorICVariant=InternalICs  ExternalResetVariant=Disabled  TRSumVariant=Passthrough  SumFdbkVariant=Disabled  SumVariant=Sum_PID  TsampFilterVariant=InternalTs  TsampNgainVariant=Passthrough  TsampIntegralVariant=Disabled_SignalSpec  ExternalSaturationOutDataTypeStr=Inherit: Same as second input
  Sum : Sum  Inputs=|++
  Sum1 : Sum  Inputs=|++
  Torque_Comparision : Scope  NumInputPorts=2
  Torque_Controlvalue : Scope  NumInputPorts=2
  dq_e(t) : Sum  Inputs=|+-
  q_e(t) : Sum  Inputs=|+-
  adjusted_torque : Outport
  wires:
  PID Controller Position/1 -> Sum/1, Torque_Controlvalue/1
  PID Controller Velocity/1 -> Torque_Controlvalue/2, Sum1/1
  dq_e(t)/1 -> PID Controller Velocity/1
  current torque/1 -> Torque_Comparision/2, Sum1/2
  q_e(t)/1 -> PID Controller Position/1
  actual position/1 -> Derivative/1, q_e(t)/2
  Sum1/1 -> Sum/2
  target position/1 -> q_e(t)/1
  Derivative/1 -> dq_e(t)/2
  Sum/1 -> Torque_Comparision/1, adjusted_torque/1
  target velocity/1 -> dq_e(t)/1

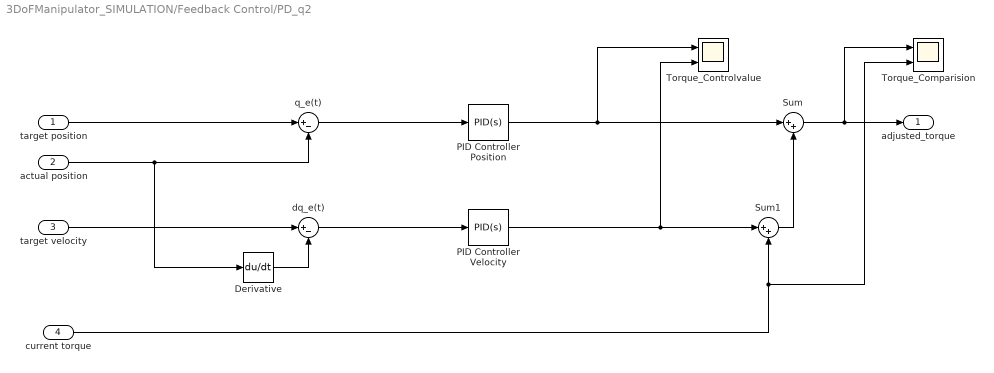
== system 3DoFManipulator_SIMULATION/Feedback Control/PD_q2 ==
  target position : Inport
  actual position : Inport  Port=2
  target velocity : Inport  Port=3
  current torque : Inport  Port=4
  Derivative : Derivative
  PID Controller Position : slpidlib/PID Controller  Controller=PID  Form=Parallel  TimeDomain=Continuous-time  UseExternalTs=off  SampleTime=-1  IntegratorMethod=Forward Euler  FilterMethod=Forward Euler  ControllerParametersSource=internal  P=300  I=0  UseKiTs=off  D=50  N=100  UseFilter=on  TunerSelectOption=Transfer Function Based (PID Tuner App)  InitialConditionSource=internal  InitialConditionForIntegrator=0  InitialConditionForFilter=0  DifferentiatorICPrevScaledInput=0  ExternalReset=none  TrackingMode=off  Kt=1  LimitOutput=off  SatLimitsSource=internal  UpperSaturationLimit=inf  LowerSaturationLimit=-inf  LinearizeAsGain=on  AntiWindupMode=none  Kb=1  LimitIntegrator=off  UpperIntegratorSaturationLimit=inf  LowerIntegratorSaturationLimit=-inf  POutMin=[]  POutMax=[]  IOutMin=[]  IOutMax=[]  DOutMin=[]  DOutMax=[]  NOutMin=[]  NOutMax=[]  SumOutMin=[]  SumOutMax=[]  SaturationOutMin=[]  SaturationOutMax=[]  PParamMin=[]  PParamMax=[]  IParamMin=[]  IParamMax=[]  DParamMin=[]  DParamMax=[]  NParamMin=[]  NParamMax=[]  KbParamMin=[]  KbParamMax=[]  KtParamMin=[]  KtParamMax=[]  KbOutMin=[]  KbOutMax=[]  KtOutMin=[]  KtOutMax=[]  IntegratorOutMin=[]  IntegratorOutMax=[]  FilterOutMin=[]  FilterOutMax=[]  SumI1OutMin=[]  SumI1OutMax=[]  SumI2OutMin=[]  SumI2OutMax=[]  SumI3OutMin=[]  SumI3OutMax=[]  SumI4OutMin=[]  SumI4OutMax=[]  SumDOutMin=[]  SumDOutMax=[]  DifferentiatorOutMin=[]  DifferentiatorOutMax=[]  FilterDiffOutCoefMin=[]  FilterDiffOutCoefMax=[]  ReciprocalOutMin=[]  ReciprocalOutMax=[]  SumDenOutMin=[]  SumDenOutMax=[]  SumNumOutMin=[]  SumNumOutMax=[]  DivideOutMin=[]  DivideOutMax=[]  UdiffTsProdOutMin=[]  UdiffTsProdOutMax=[]  NTsProdOutMin=[]  NTsProdOutMax=[]  UintegralTsProdOutMin=[]  UintegralTsProdOutMax=[]  UngainTsProdOutMin=[]  UngainTsProdOutMax=[]  ClampingZeroOutDataTypeStr=Inherit: Inherit via back propagation  ClampingZeroOutMin=[]  ClampingZeroOutMax=[]  FilterDenConstantOutDataTypeStr=Inherit: Inherit via back propagation  FilterDenConstantOutMin=[]  FilterDenConstantOutMax=[]  PCopyOutDataTypeStr=Inherit: Inherit via back propagation  PCopyOutMin=[]  PCopyOutMax=[]  NCopyOutDataTypeStr=Inherit: Inherit via back propagation  NCopyOutMin=[]  NCopyOutMax=[]  IntegratorContinuousStateAttributes=''  IntegratorStateMustResolveToSignalObject=off  IntegratorRTWStateStorageClass=Auto  FilterContinuousStateAttributes=''  FilterStateMustResolveToSignalObject=off  FilterRTWStateStorageClass=Auto  ParallelPVariant=InternalParameters  IdealPVariant=Disabled  IVariant=InternalParameters  DVariant=InternalParameters  IntegratorVariant=Continuous  SatVariant=Disabled  AWVariant=Passthrough  PCopyVariant=Disabled  TRVariant=Disabled  FdbkBlocksVariant=Forward  IdealPFdbkVariant=Disabled  SatFdbkVariant=Disabled  DerivativeFilterVariant=ContFilter  NVariant=InternalParameters  NCopyVariant=Disabled  FilterICVariant=InternalICsFilter  IntegratorICVariant=InternalICs  ExternalResetVariant=Disabled  TRSumVariant=Passthrough  SumFdbkVariant=Disabled  SumVariant=Sum_PID  TsampFilterVariant=InternalTs  TsampNgainVariant=Passthrough  TsampIntegralVariant=Disabled_SignalSpec  ExternalSaturationOutDataTypeStr=Inherit: Same as second input
  PID Controller Velocity : slpidlib/PID Controller  Controller=PID  Form=Parallel  TimeDomain=Continuous-time  UseExternalTs=off  SampleTime=-1  IntegratorMethod=Forward Euler  FilterMethod=Forward Euler  ControllerParametersSource=internal  P=10  I=0  UseKiTs=off  D=1  N=100  UseFilter=on  TunerSelectOption=Transfer Function Based (PID Tuner App)  InitialConditionSource=internal  InitialConditionForIntegrator=0  InitialConditionForFilter=0  DifferentiatorICPrevScaledInput=0  ExternalReset=none  TrackingMode=off  Kt=1  LimitOutput=off  SatLimitsSource=internal  UpperSaturationLimit=inf  LowerSaturationLimit=-inf  LinearizeAsGain=on  AntiWindupMode=none  Kb=1  LimitIntegrator=off  UpperIntegratorSaturationLimit=inf  LowerIntegratorSaturationLimit=-inf  POutMin=[]  POutMax=[]  IOutMin=[]  IOutMax=[]  DOutMin=[]  DOutMax=[]  NOutMin=[]  NOutMax=[]  SumOutMin=[]  SumOutMax=[]  SaturationOutMin=[]  SaturationOutMax=[]  PParamMin=[]  PParamMax=[]  IParamMin=[]  IParamMax=[]  DParamMin=[]  DParamMax=[]  NParamMin=[]  NParamMax=[]  KbParamMin=[]  KbParamMax=[]  KtParamMin=[]  KtParamMax=[]  KbOutMin=[]  KbOutMax=[]  KtOutMin=[]  KtOutMax=[]  IntegratorOutMin=[]  IntegratorOutMax=[]  FilterOutMin=[]  FilterOutMax=[]  SumI1OutMin=[]  SumI1OutMax=[]  SumI2OutMin=[]  SumI2OutMax=[]  SumI3OutMin=[]  SumI3OutMax=[]  SumI4OutMin=[]  SumI4OutMax=[]  SumDOutMin=[]  SumDOutMax=[]  DifferentiatorOutMin=[]  DifferentiatorOutMax=[]  FilterDiffOutCoefMin=[]  FilterDiffOutCoefMax=[]  ReciprocalOutMin=[]  ReciprocalOutMax=[]  SumDenOutMin=[]  SumDenOutMax=[]  SumNumOutMin=[]  SumNumOutMax=[]  DivideOutMin=[]  DivideOutMax=[]  UdiffTsProdOutMin=[]  UdiffTsProdOutMax=[]  NTsProdOutMin=[]  NTsProdOutMax=[]  UintegralTsProdOutMin=[]  UintegralTsProdOutMax=[]  UngainTsProdOutMin=[]  UngainTsProdOutMax=[]  ClampingZeroOutDataTypeStr=Inherit: Inherit via back propagation  ClampingZeroOutMin=[]  ClampingZeroOutMax=[]  FilterDenConstantOutDataTypeStr=Inherit: Inherit via back propagation  FilterDenConstantOutMin=[]  FilterDenConstantOutMax=[]  PCopyOutDataTypeStr=Inherit: Inherit via back propagation  PCopyOutMin=[]  PCopyOutMax=[]  NCopyOutDataTypeStr=Inherit: Inherit via back propagation  NCopyOutMin=[]  NCopyOutMax=[]  IntegratorContinuousStateAttributes=''  IntegratorStateMustResolveToSignalObject=off  IntegratorRTWStateStorageClass=Auto  FilterContinuousStateAttributes=''  FilterStateMustResolveToSignalObject=off  FilterRTWStateStorageClass=Auto  ParallelPVariant=InternalParameters  IdealPVariant=Disabled  IVariant=InternalParameters  DVariant=InternalParameters  IntegratorVariant=Continuous  SatVariant=Disabled  AWVariant=Passthrough  PCopyVariant=Disabled  TRVariant=Disabled  FdbkBlocksVariant=Forward  IdealPFdbkVariant=Disabled  SatFdbkVariant=Disabled  DerivativeFilterVariant=ContFilter  NVariant=InternalParameters  NCopyVariant=Disabled  FilterICVariant=InternalICsFilter  IntegratorICVariant=InternalICs  ExternalResetVariant=Disabled  TRSumVariant=Passthrough  SumFdbkVariant=Disabled  SumVariant=Sum_PID  TsampFilterVariant=InternalTs  TsampNgainVariant=Passthrough  TsampIntegralVariant=Disabled_SignalSpec  ExternalSaturationOutDataTypeStr=Inherit: Same as second input
  Sum : Sum  Inputs=|++
  Sum1 : Sum  Inputs=|++
  Torque_Comparision : Scope  NumInputPorts=2
  Torque_Controlvalue : Scope  NumInputPorts=2
  dq_e(t) : Sum  Inputs=|+-
  q_e(t) : Sum  Inputs=|+-
  adjusted_torque : Outport
  wires:
  PID Controller Position/1 -> Sum/1, Torque_Controlvalue/1
  PID Controller Velocity/1 -> Torque_Controlvalue/2, Sum1/1
  dq_e(t)/1 -> PID Controller Velocity/1
  current torque/1 -> Torque_Comparision/2, Sum1/2
  q_e(t)/1 -> PID Controller Position/1
  actual position/1 -> Derivative/1, q_e(t)/2
  Sum1/1 -> Sum/2
  target position/1 -> q_e(t)/1
  Derivative/1 -> dq_e(t)/2
  Sum/1 -> Torque_Comparision/1, adjusted_torque/1
  target velocity/1 -> dq_e(t)/1

== matlab function 3DoFManipulator_SIMULATION/Forward Control // Inverse Dynamic/INVERSE_DYNAMICS_BLOCK ==
  data: b0 input; tau0 output; b1 input; b2 input; ddq0 input; ddq1 input; ddq2 input; dq0 input; dq1 input; dq2 input; g input; l1 input; l2 input; m0 input; m1 input; m2 input; q1 input; q2 input; r0 input; r1 input; r2 input; tau1 output; tau2 output
function [tau0,tau1,tau2] = INVERSE_DYNAMICS_BLOCK(b0,b1,b2,ddq0,ddq1,ddq2,dq0,dq1,dq2,g,l1,l2,m0,m1,m2,q1,q2,r0,r1,r2)
%#codegen

%    This function was generated by the Symbolic Math Toolbox version 23.2.
%    20-Feb-2024 15:14:27

% b0 = complex(b0);  % if required to enforce complex operations
% b1 = complex(b1);  % if required to enforce complex operations
% b2 = complex(b2);  % if required to enforce complex operations
% ddq0 = complex(ddq0);  % if required to enforce complex operations
% ddq1 = complex(ddq1);  % if required to enforce complex operations
% ddq2 = complex(ddq2);  % if required to enforce complex operations
% dq0 = complex(dq0);  % if required to enforce complex operations
% dq1 = complex(dq1);  % if required to enforce complex operations
% dq2 = complex(dq2);  % if required to enforce complex operations
% g = complex(g);  % if required to enforce complex operations
% l1 = complex(l1);  % if required to enforce complex operations
% l2 = complex(l2);  % if required to enforce complex operations
% m0 = complex(m0);  % if required to enforce complex operations
% m1 = complex(m1);  % if required to enforce complex operations
% m2 = complex(m2);  % if required to enforce complex operations
% q1 = complex(q1);  % if required to enforce complex operations
% q2 = complex(q2);  % if required to enforce complex operations
% r0 = complex(r0);  % if required to enforce complex operations
% r1 = complex(r1);  % if required to enforce complex operations
% r2 = complex(r2);  % if required to enforce complex operations
et1 = b0.*dq0+(ddq0.*m0.*r0.^2)./2.0+ddq0.*m1.*r1.^2.*(3.0./8.0)+ddq0.*m2.*r2.^2.*(3.0./8.0)+(ddq0.*l1.^2.*m1)./6.0+(ddq0.*l1.^2.*m2)./2.0+(ddq0.*l2.^2.*m2)./6.0+(ddq0.*l1.^2.*m1.*cos(q1.*2.0))./1.2e+1+(ddq0.*l1.^2.*m2.*cos(q1.*2.0))./2.0+(ddq0.*m1.*r1.^2.*cos(q1.*2.0))./8.0+(ddq0.*l2.^2.*m2.*cos(q1.*2.0+q2.*2.0))./1.2e+1+(ddq0.*m2.*r2.^2.*cos(q1.*2.0+q2.*2.0))./8.0+(ddq0.*l1.*l2.*m2.*cos(q1.*2.0+q2))./2.0-(dq0.*dq1.*l1.^2.*m1.*sin(q1.*2.0))./6.0-dq0.*dq1.*l1.^2.*m2.*sin(q1.*2.0)-(dq0.*dq1.*m1.*r1.^2.*sin(q1.*2.0))./4.0;
et2 = dq0.*dq1.*l2.^2.*m2.*sin(q1.*2.0+q2.*2.0).*(-1.0./6.0)-(dq0.*dq2.*l2.^2.*m2.*sin(q1.*2.0+q2.*2.0))./6.0-(dq0.*dq1.*m2.*r2.^2.*sin(q1.*2.0+q2.*2.0))./4.0-(dq0.*dq2.*m2.*r2.^2.*sin(q1.*2.0+q2.*2.0))./4.0+(ddq0.*l1.*l2.*m2.*cos(q2))./2.0-(dq0.*dq2.*l1.*l2.*m2.*sin(q2))./2.0-dq0.*dq1.*l1.*l2.*m2.*sin(q1.*2.0+q2)-(dq0.*dq2.*l1.*l2.*m2.*sin(q1.*2.0+q2))./2.0;
tau0 = et1+et2;
if nargout > 1
    et3 = b1.*dq1+(ddq1.*m1.*r1.^2)./4.0+(ddq1.*m2.*r2.^2)./4.0+(ddq2.*m2.*r2.^2)./4.0+(ddq1.*l1.^2.*m1)./3.0+ddq1.*l1.^2.*m2+(ddq1.*l2.^2.*m2)./3.0+(ddq2.*l2.^2.*m2)./3.0+(g.*l2.*m2.*cos(q1+q2))./2.0+(g.*l1.*m1.*cos(q1))./2.0+g.*l1.*m2.*cos(q1)+(dq0.^2.*l1.^2.*m1.*sin(q1.*2.0))./1.2e+1+(dq0.^2.*l1.^2.*m2.*sin(q1.*2.0))./2.0+(dq0.^2.*m1.*r1.^2.*sin(q1.*2.0))./8.0+(dq0.^2.*l2.^2.*m2.*sin(q1.*2.0+q2.*2.0))./1.2e+1+(dq0.^2.*m2.*r2.^2.*sin(q1.*2.0+q2.*2.0))./8.0-(dq2.^2.*l1.*l2.*m2.*sin(q2))./2.0;
    et4 = (dq0.^2.*l1.*l2.*m2.*sin(q1.*2.0+q2))./2.0+ddq1.*l1.*l2.*m2.*cos(q2)+(ddq2.*l1.*l2.*m2.*cos(q2))./2.0-dq1.*dq2.*l1.*l2.*m2.*sin(q2);
    tau1 = et3+et4;
end
if nargout > 2
    tau2 = b2.*dq2+(ddq1.*m2.*r2.^2)./4.0+(ddq2.*m2.*r2.^2)./4.0+(ddq1.*l2.^2.*m2)./3.0+(ddq2.*l2.^2.*m2)./3.0+(g.*l2.*m2.*cos(q1+q2))./2.0+(dq0.^2.*l2.^2.*m2.*sin(q1.*2.0+q2.*2.0))./1.2e+1+(dq0.^2.*m2.*r2.^2.*sin(q1.*2.0+q2.*2.0))./8.0+(dq0.^2.*l1.*l2.*m2.*sin(q2))./4.0+(dq1.^2.*l1.*l2.*m2.*sin(q2))./2.0+(dq0.^2.*l1.*l2.*m2.*sin(q1.*2.0+q2))./4.0+(ddq1.*l1.*l2.*m2.*cos(q2))./2.0;
end
end
